simulink model "Rotating"  (R2023a)
settings: Solver=VariableStepAuto  StartTime=0.0  StopTime=40  RelTol=1e-3
values from neighbouring files (symbols this model uses):
  Kd = 0.5    [FFFB_PosForce_ME.m]    (also in FFFB_PosForce_ME1.m = 2.8284; FFFB_PosForce_ME2.m = 2.8284; FFFB_Posarbitary_actual_Mass.m = 2.8284; FFFB_arbitary_actual_Mass.m = 2.8284)
  Ki = 0.1    [FFFB_PosForce_ME.m]
  Kp = 16    [FFFB_PosForce_ME.m]    (also in FFFB_PosForce_ME1.m = 2; FFFB_PosForce_ME2.m = 2; FFFB_Posarbitary_actual_Mass.m = 2; FFFB_arbitary_actual_Mass.m = 2)
  N = [-y1+y3;-x3+x1]    [Contact.m]
  X = 0.65    [Contact.m]    (also in FFFB_PosForce_ME.m = [X0',X1',X2']; FFFB_PosForce_ME1.m = [X2']; FFFB_PosForce_ME2.m = [X110,X2']; FFFB_Posarbitary_actual_Mass.m = [X110])
  Y = [Y0',Y1',Y2']    [FFFB_PosForce_ME.m]    (also in FFFB_PosForce_ME1.m = [Y2']; FFFB_PosForce_ME2.m = [Y110,Y2']; FFFB_Posarbitary_actual_Mass.m = [Y110]; FFFB_arbitary_actual_Mass.m = [Y2'])
undefined symbols (not defined in the file or in its folder): Z
libraries: sm_lib x24, nesl_utility x8, robotcorelib x1
settings Model: Creator=91996  LastModifiedBy=91996

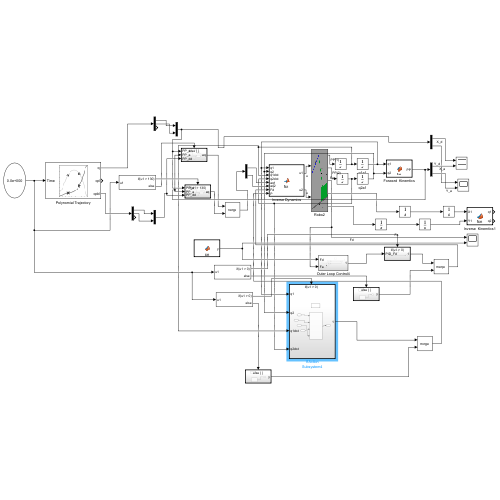
[thumbnail: Simulink's stored preview of the top-level diagram]
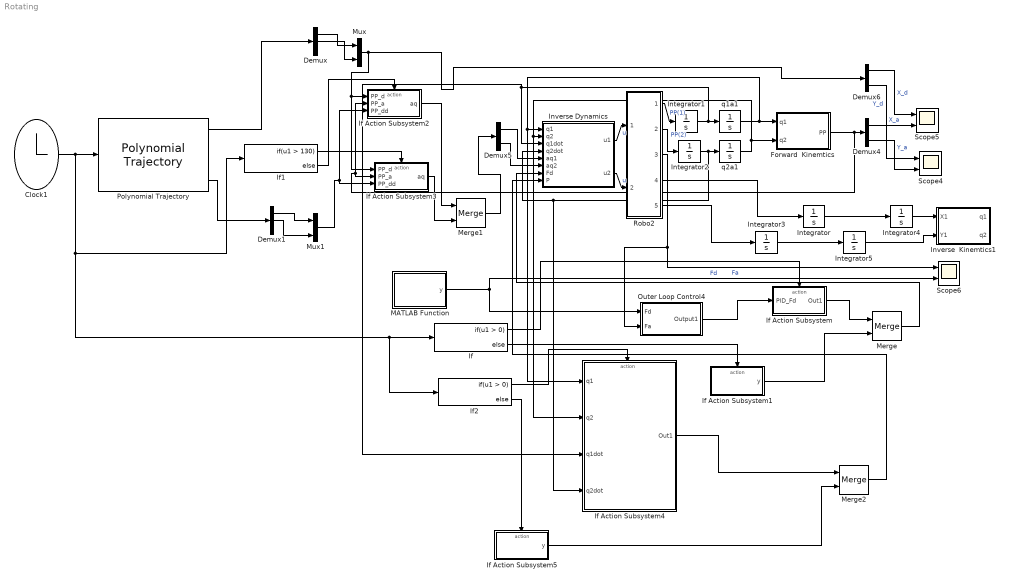
== system Rotating ==
  Clock1 : Clock
  Demux : Demux  Outputs=3
  Demux1 : Demux  Outputs=3
  Demux4 : Demux  Outputs=2
  Demux5 : Demux  Outputs=2
  Demux6 : Demux  Outputs=2
  Forward  Kinemtics : MATLAB Function  TreatAsAtomicUnit=on
  If : If
  If Action Subsystem : Subsystem  TreatAsAtomicUnit=on
  If Action Subsystem1 : Subsystem  TreatAsAtomicUnit=on
  If Action Subsystem2 : Subsystem  TreatAsAtomicUnit=on
  If Action Subsystem3 : Subsystem  TreatAsAtomicUnit=on
  If Action Subsystem4 : Subsystem  TreatAsAtomicUnit=on
  If Action Subsystem5 : Subsystem  TreatAsAtomicUnit=on
  If1 : If  IfExpression=u1 > 130
  If2 : If
  Integrator{,1..5} (6 alike) : Integrator
  Inverse  Kinemtics1 : MATLAB Function  TreatAsAtomicUnit=on
  Inverse Dynamics : MATLAB Function  TreatAsAtomicUnit=on
  MATLAB Function : MATLAB Function  TreatAsAtomicUnit=on
  Merge : Merge
  Merge1 : Merge
  Merge2 : Merge
  Mux : Mux  Inputs=2
  Mux1 : Mux  Inputs=2
  Outer Loop Control4 : Subsystem
  Polynomial Trajectory : robotcorelib/Polynomial Trajectory  WaypointSource=Internal  Waypoints=P  TimePoints=T  TimeInterval=[ 1, 4 ]  Method=Quintic Polynomial  ParameterSource=Internal  VelocityBoundaryCondition=Pd  AccelerationBoundaryCondition=Pdd  SimulateUsing=Interpreted execution
  Robo2 : Subsystem
      mask Display: image('C:\Users\91996\Desktop\2R-Robot Manipultor.png'); % Use "Edit Image" on toolstrip to change.
  Scope4 : Scope  NumInputPorts=2
  Scope5 : Scope  NumInputPorts=2
  Scope6 : Scope  NumInputPorts=2
  q1a1 : Integrator  InitialCondition=0.3330
  q2a1 : Integrator  InitialCondition=-1.5195
  wires:
  Inverse Dynamics/1(u1) -> Robo2/1(Input)  "u"
  Polynomial Trajectory/1 -> Demux/1
  Demux5/2 -> Inverse Dynamics/6(aq2)
  Demux6/2 -> Scope4/1  "Y_d"
  Mux/1 -> If Action Subsystem3/1(PP_d), If Action Subsystem2/1(PP_d), Demux6/1
  Demux1/2 -> Mux1/2
  Integrator4/1 -> Inverse  Kinemtics1/1(X1)
  Robo2/5(Y_dd) -> Integrator3/1
  Demux/1 -> Mux/1
  Integrator/1 -> Integrator4/1
  If2/1 -> If Action Subsystem4/Action
  Integrator3/1 -> Integrator5/1
  Demux1/1 -> Mux1/1
  Integrator5/1 -> Inverse  Kinemtics1/2(Y1)
  Demux5/1 -> Inverse Dynamics/5(aq1)
  Mux1/1 -> If Action Subsystem2/3(PP_dd), If Action Subsystem3/3(PP_dd)
  Polynomial Trajectory/3 -> Demux1/1
  If1/2 -> If Action Subsystem2/Action
  Demux4/1 -> Scope5/2  "X_a"
  Robo2/3(Output2) -> Scope6/1, Outer Loop Control4/2(Fa)  "Fa"
  If/1 -> If Action Subsystem/Action
  If Action Subsystem2/1(aq) -> Merge1/1
  If1/1 -> If Action Subsystem3/Action
  If Action Subsystem/1(Out1) -> Merge/1
  Merge1/1 -> Demux5/1
  Clock1/1 -> Polynomial Trajectory/1, If1/1, If2/1, If/1
  q2a1/1 -> If Action Subsystem4/2(q2), Inverse Dynamics/2(q2), Forward  Kinemtics/2(q2)
  Outer Loop Control4/1(Output1) -> If Action Subsystem/1(PID_Fd)
  If Action Subsystem3/1(aq) -> Merge1/2
  Forward  Kinemtics/1(PP) -> If Action Subsystem3/2(PP_a), If Action Subsystem2/2(PP_a), Demux4/1
  If Action Subsystem5/1(y) -> Merge2/2
  Merge2/1 -> Inverse Dynamics/8(P)
  MATLAB Function/1(y) -> Scope6/2, Outer Loop Control4/1(Fd)  "Fd"
  Robo2/4(X_dd) -> Integrator/1
  Merge/1 -> Inverse Dynamics/7(Fd)
  Integrator2/1 -> Inverse Dynamics/4(q2dot), If Action Subsystem4/4(q2dot), q2a1/1
  If Action Subsystem4/1(Out1) -> Merge2/1
  If2/2 -> If Action Subsystem5/Action
  Demux6/1 -> Scope5/1  "X_d"
  Inverse Dynamics/2(u2) -> Robo2/2(Input1)  "u"
  Integrator1/1 -> If Action Subsystem4/3(q1dot), Inverse Dynamics/3(q1dot), q1a1/1
  Robo2/2(q2_dd) -> Integrator2/1  "PP(2)"
  q1a1/1 -> Forward  Kinemtics/1(q1), If Action Subsystem4/1(q1), Inverse Dynamics/1(q1)
  Robo2/1(q1_dd) -> Integrator1/1  "PP(1)"
  If/2 -> If Action Subsystem1/Action
  Demux/2 -> Mux/2
  Demux4/2 -> Scope4/2  "Y_a"
  If Action Subsystem1/1(y) -> Merge/2

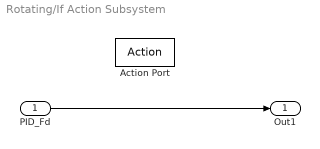
== system Rotating/If Action Subsystem ==
  PID_Fd : Inport
  Action Port : ActionPort  ActionPortLabel=if(u1 > 0)
  Out1 : Outport
  wires:
  PID_Fd/1 -> Out1/1

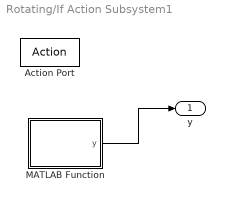
== system Rotating/If Action Subsystem1 ==
  Action Port : ActionPort  ActionPortLabel=else
  MATLAB Function : MATLAB Function  TreatAsAtomicUnit=on
  y : Outport
  wires:
  MATLAB Function/1(y) -> y/1

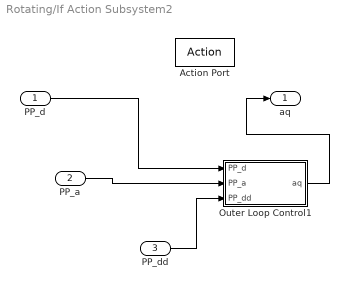
== system Rotating/If Action Subsystem2 ==
  PP_d : Inport
  PP_a : Inport  Port=2
  PP_dd : Inport  Port=3
  Action Port : ActionPort  ActionPortLabel=else
  Outer Loop Control1 : Subsystem
  aq : Outport
  wires:
  PP_d/1 -> Outer Loop Control1/1(PP_d)
  PP_dd/1 -> Outer Loop Control1/3(PP_dd)
  Outer Loop Control1/1(aq) -> aq/1
  PP_a/1 -> Outer Loop Control1/2(PP_a)

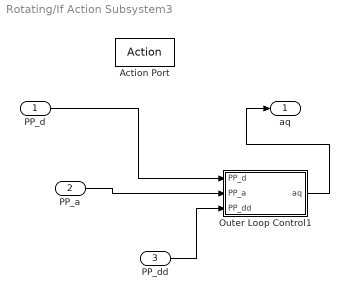
== system Rotating/If Action Subsystem3 ==
  PP_d : Inport
  PP_a : Inport  Port=2
  PP_dd : Inport  Port=3
  Action Port : ActionPort  ActionPortLabel=if(u1 > 130)
  Outer Loop Control1 : Subsystem
  aq : Outport
  wires:
  Outer Loop Control1/1(aq) -> aq/1
  PP_dd/1 -> Outer Loop Control1/3(PP_dd)
  PP_a/1 -> Outer Loop Control1/2(PP_a)
  PP_d/1 -> Outer Loop Control1/1(PP_d)

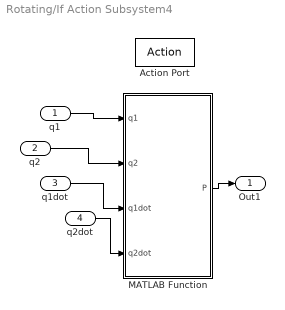
== system Rotating/If Action Subsystem4 ==
  q1 : Inport
  q2 : Inport  Port=2
  q1dot : Inport  Port=3
  q2dot : Inport  Port=4
  Action Port : ActionPort  ActionPortLabel=if(u1 > 0)
  MATLAB Function : MATLAB Function  TreatAsAtomicUnit=on
  Out1 : Outport
  wires:
  MATLAB Function/1(P) -> Out1/1
  q1/1 -> MATLAB Function/1(q1)
  q2/1 -> MATLAB Function/2(q2)
  q1dot/1 -> MATLAB Function/3(q1dot)
  q2dot/1 -> MATLAB Function/4(q2dot)

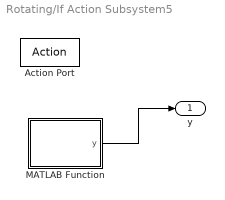
== system Rotating/If Action Subsystem5 ==
  Action Port : ActionPort  ActionPortLabel=else
  MATLAB Function : MATLAB Function  TreatAsAtomicUnit=on
  y : Outport
  wires:
  MATLAB Function/1(y) -> y/1

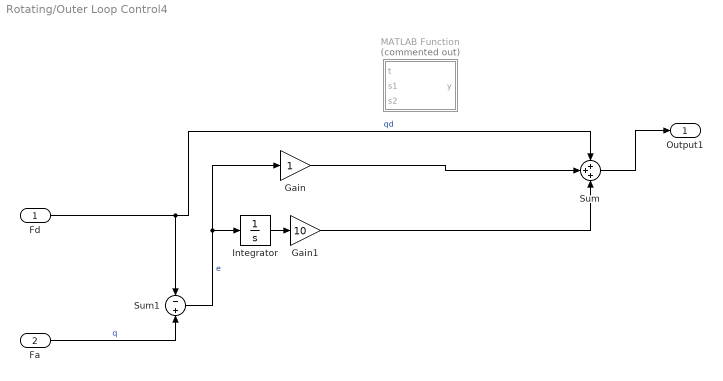
== system Rotating/Outer Loop Control4 ==
  Fd : Inport
  Fa : Inport  Port=2
  Gain : Gain
  Gain1 : Gain  Gain=10
  Integrator : Integrator
  MATLAB Function : MATLAB Function  Commented=on  TreatAsAtomicUnit=on
  Sum : Sum  Inputs=+++
  Sum1 : Sum  Inputs=-+
  Output1 : Outport
  wires:
  Sum1/1 -> Gain/1, Integrator/1  "e"
  Fd/1 -> Sum/1, Sum1/1  "qd"
  Fa/1 -> Sum1/2  "q"
  Integrator/1 -> Gain1/1
  Gain/1 -> Sum/2
  Gain1/1 -> Sum/3
  Sum/1 -> Output1/1

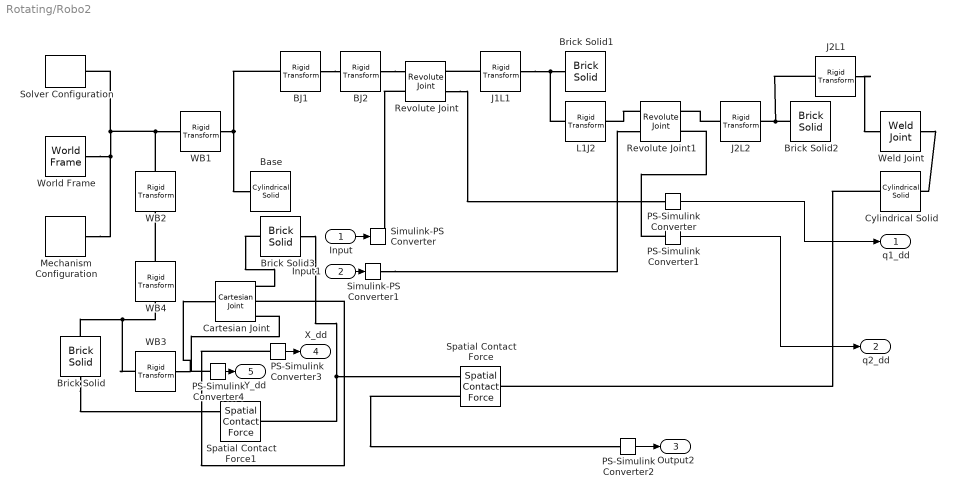
== system Rotating/Robo2 ==
  Input : Inport
  Input1 : Inport  Port=2
  BJ1 : sm_lib/Frames and Transforms/Rigid Transform  TranslationMethod=StandardAxis  TranslationStandardOffset=0.25  TranslationStandardOffsetUnits=m  TranslationStandardAxis=+Z  TranslationCartesianOffset=[0 0 0]  TranslationCartesianOffsetUnits=m  TranslationROffset=0  TranslationROffsetUnits=m  TranslationZOffset=0  TranslationZOffsetUnits=m  TranslationThetaOffset=0  TranslationThetaOffsetUnits=deg  RotationMethod=StandardAxis  RotationAngleUnits=deg  RotationStandardAxis=+X  RotationAngle=90  RotationArbitraryAxis=[0 0 1]  FollAlignAxisA=+X  BaseAlignAxisA=+Y  FollAlignAxisB=+Y  BaseAlignAxisB=+Z  RotationSequenceAxes=FollowerAxes  RotationSequence=XYX  RotationSequenceAngles=[0 0 0]  RotationSequenceAnglesUnits=deg  RotationMatrix=[1 0 0; 0 1 0; 0 0 1]  Quaternion=[1 0 0 0]
  BJ2 : sm_lib/Frames and Transforms/Rigid Transform  TranslationMethod=None  TranslationStandardOffset=0  TranslationStandardOffsetUnits=m  TranslationStandardAxis=+Z  TranslationCartesianOffset=[0 0 0]  TranslationCartesianOffsetUnits=m  TranslationROffset=0  TranslationROffsetUnits=m  TranslationZOffset=0  TranslationZOffsetUnits=m  TranslationThetaOffset=0  TranslationThetaOffsetUnits=deg  RotationMethod=StandardAxis  RotationAngleUnits=rad  RotationStandardAxis=+Z  RotationAngle=0.3330  RotationArbitraryAxis=[0 0 1]  FollAlignAxisA=+X  BaseAlignAxisA=+Y  FollAlignAxisB=+Y  BaseAlignAxisB=+Z  RotationSequenceAxes=FollowerAxes  RotationSequence=XYX  RotationSequenceAngles=[0 0 0]  RotationSequenceAnglesUnits=deg  RotationMatrix=[1 0 0; 0 1 0; 0 0 1]  Quaternion=[1 0 0 0]
  Base : sm_lib/Body Elements/Cylindrical Solid  GraphicAmbientColor=[0.15 0.15 0.15 1.0]  BasedOnType=Density  CenterOfMass=[0 0 0]  CenterOfMassUnits=m  GraphicDiffuseColor=[0.5 0.5 0.5]  CylinderLength=0.5  CylinderLengthUnits=m  CylinderRadius=0.02  CylinderRadiusUnits=m  Density=10000  DensityUnits=kg/m^3  DoExposeReferenceFrame=on  GraphicEmissiveColor=[0.0 0.0 0.0 1.0]  ExportEntireGeometry=off  SerializedFrames=<Frames/>  MarkerShape=Sphere  MarkerSize=10  GraphicType=FromGeometry  InertiaType=CalculateFromGeometry  Mass=1  MassUnits=kg  MomentsOfInertia=[1 1 1]  MomentsOfInertiaUnits=kg*m^2  GraphicOpacity=1.0  ProductsOfInertia=[0 0 0]  ProductsOfInertiaUnits=kg*m^2  GraphicShininess=75  GraphicSpecularColor=[0.5 0.5 0.5 1.0]  GraphicVisPropType=SimpleVisualProperties
  Brick Solid : sm_lib/Body Elements/Brick Solid  GraphicAmbientColor=[0.15 0.15 0.15 1.0]  BasedOnType=Density  BrickDimensions=[1 0.02 0.02]  BrickDimensionsUnits=m  CenterOfMass=[0 0 0]  CenterOfMassUnits=m  GraphicDiffuseColor=[0.5 0.5 0.5]  Density=10000  DensityUnits=kg/m^3  DoExposeReferenceFrame=on  GraphicEmissiveColor=[0.0 0.0 0.0 1.0]  ExportEntireGeometry=on  SerializedFrames=<Frames/>  MarkerShape=Sphere  MarkerSize=10  GraphicType=FromGeometry  InertiaType=CalculateFromGeometry  Mass=1  MassUnits=kg  MomentsOfInertia=[1 1 1]  MomentsOfInertiaUnits=kg*m^2  GraphicOpacity=1.0  ProductsOfInertia=[0 0 0]  ProductsOfInertiaUnits=kg*m^2  GraphicShininess=75  GraphicSpecularColor=[0.5 0.5 0.5 1.0]  GraphicVisPropType=SimpleVisualProperties
  Brick Solid1 : sm_lib/Body Elements/Brick Solid  GraphicAmbientColor=[0.15 0.15 0.15 1.0]  BasedOnType=Density  BrickDimensions=[0.5 0.02 0.02]  BrickDimensionsUnits=m  CenterOfMass=[0 0 0]  CenterOfMassUnits=m  GraphicDiffuseColor=[0.2 0.2 1.0]  Density=7800  DensityUnits=kg/m^3  DoExposeReferenceFrame=on  GraphicEmissiveColor=[0.0 0.0 0.0 1.0]  ExportEntireGeometry=off  SerializedFrames=<Frames/>  MarkerShape=Sphere  MarkerSize=10  GraphicType=FromGeometry  InertiaType=CalculateFromGeometry  Mass=1  MassUnits=kg  MomentsOfInertia=[1 1 1]  MomentsOfInertiaUnits=kg*m^2  GraphicOpacity=1.0  ProductsOfInertia=[0 0 0]  ProductsOfInertiaUnits=kg*m^2  GraphicShininess=75  GraphicSpecularColor=[0.5 0.5 0.5 1.0]  GraphicVisPropType=SimpleVisualProperties
  Brick Solid2 : sm_lib/Body Elements/Brick Solid  GraphicAmbientColor=[0.15 0.15 0.15 1.0]  BasedOnType=Density  BrickDimensions=[0.5-0.01 0.02 0.02]  BrickDimensionsUnits=m  CenterOfMass=[0 0 0]  CenterOfMassUnits=m  GraphicDiffuseColor=[0.0 0.8 0.2]  Density=7800  DensityUnits=kg/m^3  DoExposeReferenceFrame=on  GraphicEmissiveColor=[0.0 0.0 0.0 1.0]  ExportEntireGeometry=off  SerializedFrames=<Frames/>  MarkerShape=Sphere  MarkerSize=10  GraphicType=FromGeometry  InertiaType=CalculateFromGeometry  Mass=1  MassUnits=kg  MomentsOfInertia=[1 1 1]  MomentsOfInertiaUnits=kg*m^2  GraphicOpacity=1.0  ProductsOfInertia=[0 0 0]  ProductsOfInertiaUnits=kg*m^2  GraphicShininess=75  GraphicSpecularColor=[0.5 0.5 0.5 1.0]  GraphicVisPropType=SimpleVisualProperties
  Brick Solid3 : sm_lib/Body Elements/Brick Solid  GraphicAmbientColor=[0.15 0.15 0.15 1.0]  BasedOnType=Density  BrickDimensions=[0.2 0.02 0.2]  BrickDimensionsUnits=m  CenterOfMass=[0 0 0]  CenterOfMassUnits=m  GraphicDiffuseColor=[0.5 0.5 0.5]  Density=2000  DensityUnits=kg/m^3  DoExposeReferenceFrame=on  GraphicEmissiveColor=[0.0 0.0 0.0 1.0]  ExportEntireGeometry=on  SerializedFrames=<Frames/>  MarkerShape=Sphere  MarkerSize=10  GraphicType=FromGeometry  InertiaType=CalculateFromGeometry  Mass=1  MassUnits=kg  MomentsOfInertia=[1 1 1]  MomentsOfInertiaUnits=kg*m^2  GraphicOpacity=1.0  ProductsOfInertia=[0 0 0]  ProductsOfInertiaUnits=kg*m^2  GraphicShininess=75  GraphicSpecularColor=[0.5 0.5 0.5 1.0]  GraphicVisPropType=SimpleVisualProperties
  Cartesian Joint : sm_lib/Joints/Cartesian Joint  JointMode=Normal  SenseConstraintForce=off  SenseConstraintForceX=off  SenseConstraintForceY=off  SenseConstraintForceZ=off  SenseConstraintTorque=off  SenseConstraintTorqueX=off  SenseConstraintTorqueY=off  SenseConstraintTorqueZ=off  SenseTotalForce=off  SenseTotalForceX=off  SenseTotalForceY=off  SenseTotalForceZ=off  SenseTotalTorque=off  SenseTotalTorqueX=off  SenseTotalTorqueY=off  SenseTotalTorqueZ=off  CompositeWrenchDir=FollowerOnBase  CompositeWrenchFrame=BaseFrame  PxEquilibriumPosition=0  PxEquilibriumPositionUnits=m  PxSpringStiffness=0  PxSpringStiffnessUnits=N/m  PxDampingCoefficient=0  PxDampingCoefficientUnits=N/(m/s)  PxTorqueActuationMode=NoTorque  PxMotionActuationMode=ComputedMotion  PxSensePosition=off  PxSenseVelocity=off  PxSenseAcceleration=on  PxSenseTorqueForce=off  PxSenseLowerLimitTorqueForce=off  PxSenseUpperLimitTorqueForce=off  PxLowerLimitSpecify=off  PxLowerLimitBound=-1  PxLowerLimitBoundUnits=m  PxLowerLimitStiffness=1e6  PxLowerLimitStiffnessUnits=N/m  PxLowerLimitDamping=1e3  PxLowerLimitDampingUnits=N/(m/s)  PxLowerLimitTransitionRegionWidth=1e-4  PxLowerLimitTransitionRegionWidthUnits=m  PxUpperLimitSpecify=off  PxUpperLimitBound=1  PxUpperLimitBoundUnits=m  PxUpperLimitStiffness=1e6  PxUpperLimitStiffnessUnits=N/m  PxUpperLimitDamping=1e3  PxUpperLimitDampingUnits=N/(m/s)  PxUpperLimitTransitionRegionWidth=1e-4  PxUpperLimitTransitionRegionWidthUnits=m  PxPositionTargetSpecify=off  PxPositionTargetPriority=High  PxPositionTargetValue=0  PxPositionTargetValueUnits=m  PxVelocityTargetSpecify=off  PxVelocityTargetPriority=High  PxVelocityTargetValue=0  PxVelocityTargetValueUnits=m/s  PyEquilibriumPosition=0  PyEquilibriumPositionUnits=m  PySpringStiffness=0  PySpringStiffnessUnits=N/m  PyDampingCoefficient=0  PyDampingCoefficientUnits=N/(m/s)  PyTorqueActuationMode=NoTorque  PyMotionActuationMode=ComputedMotion  PySensePosition=off  PySenseVelocity=off  PySenseAcceleration=off  PySenseTorqueForce=off  PySenseLowerLimitTorqueForce=off  PySenseUpperLimitTorqueForce=off  PyLowerLimitSpecify=off  PyLowerLimitBound=-1  PyLowerLimitBoundUnits=m  PyLowerLimitStiffness=1e6  PyLowerLimitStiffnessUnits=N/m  PyLowerLimitDamping=1e3  PyLowerLimitDampingUnits=N/(m/s)  PyLowerLimitTransitionRegionWidth=1e-4  PyLowerLimitTransitionRegionWidthUnits=m  PyUpperLimitSpecify=off  PyUpperLimitBound=1  PyUpperLimitBoundUnits=m  PyUpperLimitStiffness=1e6  PyUpperLimitStiffnessUnits=N/m  PyUpperLimitDamping=1e3  PyUpperLimitDampingUnits=N/(m/s)  PyUpperLimitTransitionRegionWidth=1e-4  PyUpperLimitTransitionRegionWidthUnits=m  PyPositionTargetSpecify=off  PyPositionTargetPriority=High  PyPositionTargetValue=0  PyPositionTargetValueUnits=m  PyVelocityTargetSpecify=off  PyVelocityTargetPriority=High  PyVelocityTargetValue=0  PyVelocityTargetValueUnits=m/s  PzEquilibriumPosition=0  PzEquilibriumPositionUnits=m  PzSpringStiffness=0  PzSpringStiffnessUnits=N/m  PzDampingCoefficient=0  PzDampingCoefficientUnits=N/(m/s)  PzTorqueActuationMode=NoTorque  PzMotionActuationMode=ComputedMotion  PzSensePosition=off  PzSenseVelocity=off  PzSenseAcceleration=on  PzSenseTorqueForce=off  PzSenseLowerLimitTorqueForce=off  PzSenseUpperLimitTorqueForce=off  PzLowerLimitSpecify=off  PzLowerLimitBound=-1  PzLowerLimitBoundUnits=m  PzLowerLimitStiffness=1e6  PzLowerLimitStiffnessUnits=N/m  PzLowerLimitDamping=1e3  PzLowerLimitDampingUnits=N/(m/s)  PzLowerLimitTransitionRegionWidth=1e-4  PzLowerLimitTransitionRegionWidthUnits=m  PzUpperLimitSpecify=off  PzUpperLimitBound=1  PzUpperLimitBoundUnits=m  PzUpperLimitStiffness=1e6  PzUpperLimitStiffnessUnits=N/m  PzUpperLimitDamping=1e3  PzUpperLimitDampingUnits=N/(m/s)  PzUpperLimitTransitionRegionWidth=1e-4  PzUpperLimitTransitionRegionWidthUnits=m  PzPositionTargetSpecify=off  PzPositionTargetPriority=High  PzPositionTargetValue=0  PzPositionTargetValueUnits=m  PzVelocityTargetSpecify=off  PzVelocityTargetPriority=High  PzVelocityTargetValue=0  PzVelocityTargetValueUnits=m/s
  Cylindrical Solid : sm_lib/Body Elements/Cylindrical Solid  GraphicAmbientColor=[0.15 0.15 0.15 1.0]  BasedOnType=Density  CenterOfMass=[0 0 0]  CenterOfMassUnits=m  GraphicDiffuseColor=[0.5 0.5 0.5]  CylinderLength=0.02  CylinderLengthUnits=m  CylinderRadius=0.01  CylinderRadiusUnits=m  Density=7800  DensityUnits=kg/m^3  DoExposeReferenceFrame=on  GraphicEmissiveColor=[0.0 0.0 0.0 1.0]  ExportEntireGeometry=on  SerializedFrames=<Frames/>  MarkerShape=Sphere  MarkerSize=10  GraphicType=FromGeometry  InertiaType=CalculateFromGeometry  Mass=1  MassUnits=kg  MomentsOfInertia=[1 1 1]  MomentsOfInertiaUnits=kg*m^2  GraphicOpacity=1.0  ProductsOfInertia=[0 0 0]  ProductsOfInertiaUnits=kg*m^2  GraphicShininess=75  GraphicSpecularColor=[0.5 0.5 0.5 1.0]  GraphicVisPropType=SimpleVisualProperties
  J1L1 : sm_lib/Frames and Transforms/Rigid Transform  TranslationMethod=StandardAxis  TranslationStandardOffset=0.25  TranslationStandardOffsetUnits=m  TranslationStandardAxis=+X  TranslationCartesianOffset=[0 0 0]  TranslationCartesianOffsetUnits=m  TranslationROffset=0  TranslationROffsetUnits=m  TranslationZOffset=0  TranslationZOffsetUnits=m  TranslationThetaOffset=0  TranslationThetaOffsetUnits=deg  RotationMethod=None  RotationAngleUnits=deg  RotationStandardAxis=+Z  RotationAngle=0.0  RotationArbitraryAxis=[0 0 1]  FollAlignAxisA=+X  BaseAlignAxisA=+Y  FollAlignAxisB=+Y  BaseAlignAxisB=+Z  RotationSequenceAxes=FollowerAxes  RotationSequence=XYX  RotationSequenceAngles=[0 0 0]  RotationSequenceAnglesUnits=deg  RotationMatrix=[1 0 0; 0 1 0; 0 0 1]  Quaternion=[1 0 0 0]
  J2L1 : sm_lib/Frames and Transforms/Rigid Transform  TranslationMethod=StandardAxis  TranslationStandardOffset=(0.5-0.01)/2  TranslationStandardOffsetUnits=m  TranslationStandardAxis=+X  TranslationCartesianOffset=[0 0 0]  TranslationCartesianOffsetUnits=m  TranslationROffset=0  TranslationROffsetUnits=m  TranslationZOffset=0  TranslationZOffsetUnits=m  TranslationThetaOffset=0  TranslationThetaOffsetUnits=deg  RotationMethod=None  RotationAngleUnits=deg  RotationStandardAxis=+Z  RotationAngle=0.0  RotationArbitraryAxis=[0 0 1]  FollAlignAxisA=+X  BaseAlignAxisA=+Y  FollAlignAxisB=+Y  BaseAlignAxisB=+Z  RotationSequenceAxes=FollowerAxes  RotationSequence=XYX  RotationSequenceAngles=[0 0 0]  RotationSequenceAnglesUnits=deg  RotationMatrix=[1 0 0; 0 1 0; 0 0 1]  Quaternion=[1 0 0 0]
  J2L2 : sm_lib/Frames and Transforms/Rigid Transform  TranslationMethod=StandardAxis  TranslationStandardOffset=(0.5-0.01)/2  TranslationStandardOffsetUnits=m  TranslationStandardAxis=+X  TranslationCartesianOffset=[0 0 0]  TranslationCartesianOffsetUnits=m  TranslationROffset=0  TranslationROffsetUnits=m  TranslationZOffset=0  TranslationZOffsetUnits=m  TranslationThetaOffset=0  TranslationThetaOffsetUnits=deg  RotationMethod=None  RotationAngleUnits=deg  RotationStandardAxis=+Z  RotationAngle=0.0  RotationArbitraryAxis=[0 0 1]  FollAlignAxisA=+X  BaseAlignAxisA=+Y  FollAlignAxisB=+Y  BaseAlignAxisB=+Z  RotationSequenceAxes=FollowerAxes  RotationSequence=XYX  RotationSequenceAngles=[0 0 0]  RotationSequenceAnglesUnits=deg  RotationMatrix=[1 0 0; 0 1 0; 0 0 1]  Quaternion=[1 0 0 0]
  L1J2 : sm_lib/Frames and Transforms/Rigid Transform  TranslationMethod=StandardAxis  TranslationStandardOffset=0.25  TranslationStandardOffsetUnits=m  TranslationStandardAxis=+X  TranslationCartesianOffset=[0 0 0]  TranslationCartesianOffsetUnits=m  TranslationROffset=0  TranslationROffsetUnits=m  TranslationZOffset=0  TranslationZOffsetUnits=m  TranslationThetaOffset=0  TranslationThetaOffsetUnits=deg  RotationMethod=StandardAxis  RotationAngleUnits=rad  RotationStandardAxis=+Z  RotationAngle=-1.5195  RotationArbitraryAxis=[0 0 1]  FollAlignAxisA=+X  BaseAlignAxisA=+Y  FollAlignAxisB=+Y  BaseAlignAxisB=+Z  RotationSequenceAxes=FollowerAxes  RotationSequence=XYX  RotationSequenceAngles=[0 0 0]  RotationSequenceAnglesUnits=deg  RotationMatrix=[1 0 0; 0 1 0; 0 0 1]  Quaternion=[1 0 0 0]
  Mechanism Configuration : sm_lib/Utilities/Mechanism Configuration  UniformGravity=Constant  GravityVector=[0 0 -9.80665]  GravityVectorUnits=m/s^2  LinearizationDelta=0.001  JointModeTransitionNonlinearIterations=2
  PS-Simulink Converter{,1..4} (5 alike) : nesl_utility/PS-Simulink Converter  PhysicalDomain=network_engine_domain  SubClassName=ps_output  LeftPortType=input  RightPortType=output  PseudoPeriodic=off  Frequencies=[]  VectorFormat=inherit  Unit=inherit  AffineConversion=off
  Revolute Joint : sm_lib/Joints/Revolute Joint  JointMode=Normal  SenseConstraintForce=off  SenseConstraintForceX=off  SenseConstraintForceY=off  SenseConstraintForceZ=off  SenseConstraintTorque=off  SenseConstraintTorqueX=off  SenseConstraintTorqueY=off  SenseConstraintTorqueZ=off  SenseTotalForce=off  SenseTotalForceX=off  SenseTotalForceY=off  SenseTotalForceZ=off  SenseTotalTorque=off  SenseTotalTorqueX=off  SenseTotalTorqueY=off  SenseTotalTorqueZ=off  CompositeWrenchDir=FollowerOnBase  CompositeWrenchFrame=BaseFrame  EquilibriumPosition=0  EquilibriumPositionUnits=deg  SpringStiffness=0  SpringStiffnessUnits=N*m/deg  DampingCoefficient=0  DampingCoefficientUnits=N*m/(deg/s)  TorqueActuationMode=InputTorque  MotionActuationMode=ComputedMotion  SensePosition=off  SenseVelocity=off  SenseAcceleration=on  SenseTorqueForce=off  SenseLowerLimitTorqueForce=off  SenseUpperLimitTorqueForce=off  LowerLimitSpecify=off  LowerLimitBound=-90  LowerLimitBoundUnits=deg  LowerLimitStiffness=1e4  LowerLimitStiffnessUnits=N*m/deg  LowerLimitDamping=10  LowerLimitDampingUnits=N*m/(deg/s)  LowerLimitTransitionRegionWidth=0.1  LowerLimitTransitionRegionWidthUnits=deg  UpperLimitSpecify=off  UpperLimitBound=90  UpperLimitBoundUnits=deg  UpperLimitStiffness=1e4  UpperLimitStiffnessUnits=N*m/deg  UpperLimitDamping=10  UpperLimitDampingUnits=N*m/(deg/s)  UpperLimitTransitionRegionWidth=0.1  UpperLimitTransitionRegionWidthUnits=deg  PositionTargetSpecify=off  PositionTargetPriority=High  PositionTargetValue=0  PositionTargetValueUnits=deg  VelocityTargetSpecify=off  VelocityTargetPriority=High  VelocityTargetValue=0  VelocityTargetValueUnits=deg/s
  Revolute Joint1 : sm_lib/Joints/Revolute Joint  JointMode=Normal  SenseConstraintForce=off  SenseConstraintForceX=off  SenseConstraintForceY=off  SenseConstraintForceZ=off  SenseConstraintTorque=off  SenseConstraintTorqueX=off  SenseConstraintTorqueY=off  SenseConstraintTorqueZ=off  SenseTotalForce=off  SenseTotalForceX=off  SenseTotalForceY=off  SenseTotalForceZ=off  SenseTotalTorque=off  SenseTotalTorqueX=off  SenseTotalTorqueY=off  SenseTotalTorqueZ=off  CompositeWrenchDir=FollowerOnBase  CompositeWrenchFrame=BaseFrame  EquilibriumPosition=0  EquilibriumPositionUnits=deg  SpringStiffness=0  SpringStiffnessUnits=N*m/deg  DampingCoefficient=0  DampingCoefficientUnits=N*m/(deg/s)  TorqueActuationMode=InputTorque  MotionActuationMode=ComputedMotion  SensePosition=off  SenseVelocity=off  SenseAcceleration=on  SenseTorqueForce=off  SenseLowerLimitTorqueForce=off  SenseUpperLimitTorqueForce=off  LowerLimitSpecify=off  LowerLimitBound=-90  LowerLimitBoundUnits=deg  LowerLimitStiffness=1e4  LowerLimitStiffnessUnits=N*m/deg  LowerLimitDamping=10  LowerLimitDampingUnits=N*m/(deg/s)  LowerLimitTransitionRegionWidth=0.1  LowerLimitTransitionRegionWidthUnits=deg  UpperLimitSpecify=off  UpperLimitBound=90  UpperLimitBoundUnits=deg  UpperLimitStiffness=1e4  UpperLimitStiffnessUnits=N*m/deg  UpperLimitDamping=10  UpperLimitDampingUnits=N*m/(deg/s)  UpperLimitTransitionRegionWidth=0.1  UpperLimitTransitionRegionWidthUnits=deg  PositionTargetSpecify=off  PositionTargetPriority=High  PositionTargetValue=0  PositionTargetValueUnits=deg  VelocityTargetSpecify=off  VelocityTargetPriority=High  VelocityTargetValue=0  VelocityTargetValueUnits=deg/s
  Simulink-PS Converter : nesl_utility/Simulink-PS Converter  PhysicalDomain=network_engine_domain  SubClassName=ps_input  LeftPortType=input  RightPortType=output  PseudoPeriodic=off  Frequencies=[]  NoiseDistribution=none  NoiseParameters=[]  Unit=N*m  AffineConversion=off  FilteringAndDerivatives=provide  SimscapeFilterOrder=1  InputFilterTimeConstant=0.001  UdotUserProvided=0
  Simulink-PS Converter1 : nesl_utility/Simulink-PS Converter  PhysicalDomain=network_engine_domain  SubClassName=ps_input  LeftPortType=input  RightPortType=output  PseudoPeriodic=off  Frequencies=[]  NoiseDistribution=none  NoiseParameters=[]  Unit=N*m  AffineConversion=off  FilteringAndDerivatives=provide  SimscapeFilterOrder=1  InputFilterTimeConstant=0.001  UdotUserProvided=0
  Solver Configuration : nesl_utility/Solver Configuration  PhysicalDomain=network_engine_domain  SubClassName=solver  LeftPortType=input  RightPortType=generic  Tones=[]  Harmonics=[]  SimulateNoise=off  Profile=off  UseLocalSampling=off  EnableSwitchedLinearOptims=on  FrequencyDomain=off  UseCCode=off  RelTol=0.001  AbsTol=1e-06  MinStep=1e-09  ToWorkspace=off  RevertToSquareIcSolve=off  NumHomotopyIterations=100  PhasorMode=off  PhasorModeNumHarmonics=1  ConsistencySolver=NEWTON_XTOL_AFTER_FTOL  IndexReductionMethod=DerivativeReplacement  DoDC=off  ResidualTolerance=1e-09  ConsistencyTolSource=GLOBAL  ConsistencyAbsTol=0.001  ConsistencyRelTol=0.001  ConsistencyTolFactor=0.001  UseLocalSolver=off  LocalSolverChoice=NE_BACKWARD_EULER_ADVANCER  ResolveIndetEquations=on  FunctionEvalNumThread=1  LocalSolverSampleTime=0.001  DoFixedCost=off  MaxNonlinIter=3  MaxModeIter=2  ComputeImpulses=off  ImpulseIterations=2  LinearAlgebra=Sparse  LinearAlgebraNumThread=0  EquationFormulation=NE_TIME_EF  DelaysMemoryBudget=1024  AutomaticFiltering=on  FilteringTimeConstant=0.001  PartitionStorageMethod=AS_NEEDED  PartitionMemoryBudget=1024  PartitionMethod=FAST
  Spatial Contact Force : sm_lib/Forces and Torques/Spatial Contact Force  SenseContactBaseRotation=off  SenseContactBaseTranslation=off  CoefficientOfDynamicFriction=0.3  CoefficientOfStaticFriction=0.5  NormalDamping=1e6  NormalDampingUnits=N/(m/s)  SenseContactSignal=off  NormalStiffness=1e6  NormalStiffnessUnits=N/m  FrictionalCriticalVelocity=1e-3  FrictionalCriticalVelocityUnits=m/s  ZeroCrossDetectContactStartAndEnd=off  SenseContactFollowerRotation=off  SenseContactFollowerTranslation=off  FrictionType=SmoothStickSlip  SenseFrictionalForceMagnitude=off  SenseNormalForceMagnitude=on  NormalForceType=SmoothSpringDamper  SenseNormalVelocity=off  SenseSeparationDistance=off  SenseTangentialVelocity=off  NormalTransitionRegionWidth=1e-4  NormalTransitionRegionWidthUnits=m
  Spatial Contact Force1 : sm_lib/Forces and Torques/Spatial Contact Force  SenseContactBaseRotation=off  SenseContactBaseTranslation=off  CoefficientOfDynamicFriction=0.05  CoefficientOfStaticFriction=0.1  NormalDamping=1e6  NormalDampingUnits=N/(m/s)  SenseContactSignal=off  NormalStiffness=1e6  NormalStiffnessUnits=N/m  FrictionalCriticalVelocity=1e-3  FrictionalCriticalVelocityUnits=m/s  ZeroCrossDetectContactStartAndEnd=off  SenseContactFollowerRotation=off  SenseContactFollowerTranslation=off  FrictionType=SmoothStickSlip  SenseFrictionalForceMagnitude=off  SenseNormalForceMagnitude=on  NormalForceType=SmoothSpringDamper  SenseNormalVelocity=off  SenseSeparationDistance=off  SenseTangentialVelocity=off  NormalTransitionRegionWidth=1e-4  NormalTransitionRegionWidthUnits=m
  WB1 : sm_lib/Frames and Transforms/Rigid Transform  TranslationMethod=Cartesian  TranslationStandardOffset=0  TranslationStandardOffsetUnits=m  TranslationStandardAxis=+Z  TranslationCartesianOffset=[0 0.25 0]  TranslationCartesianOffsetUnits=m  TranslationROffset=0  TranslationROffsetUnits=m  TranslationZOffset=0  TranslationZOffsetUnits=m  TranslationThetaOffset=0  TranslationThetaOffsetUnits=deg  RotationMethod=None  RotationAngleUnits=deg  RotationStandardAxis=+X  RotationAngle=90  RotationArbitraryAxis=[0 0 1]  FollAlignAxisA=+X  BaseAlignAxisA=+Y  FollAlignAxisB=+Y  BaseAlignAxisB=+Z  RotationSequenceAxes=FollowerAxes  RotationSequence=XYX  RotationSequenceAngles=[0 0 0]  RotationSequenceAnglesUnits=deg  RotationMatrix=[1 0 0; 0 1 0; 0 0 1]  Quaternion=[1 0 0 0]
  WB2 : sm_lib/Frames and Transforms/Rigid Transform  TranslationMethod=Cartesian  TranslationStandardOffset=0  TranslationStandardOffsetUnits=m  TranslationStandardAxis=+Z  TranslationCartesianOffset="[-0.5   -0.25  0.25 ]"  TranslationCartesianOffsetUnits=m  TranslationROffset=0  TranslationROffsetUnits=m  TranslationZOffset=0  TranslationZOffsetUnits=m  TranslationThetaOffset=0  TranslationThetaOffsetUnits=deg  RotationMethod=None  RotationAngleUnits=deg  RotationStandardAxis=+X  RotationAngle=90  RotationArbitraryAxis=[0 0 1]  FollAlignAxisA=+X  BaseAlignAxisA=+Y  FollAlignAxisB=+Y  BaseAlignAxisB=+Z  RotationSequenceAxes=FollowerAxes  RotationSequence=XYX  RotationSequenceAngles=[0 0 0]  RotationSequenceAnglesUnits=deg  RotationMatrix=[1 0 0; 0 1 0; 0 0 1]  Quaternion=[1 0 0 0]
  WB3 : sm_lib/Frames and Transforms/Rigid Transform  TranslationMethod=Cartesian  TranslationStandardOffset=0  TranslationStandardOffsetUnits=m  TranslationStandardAxis=+Z  TranslationCartesianOffset="[-0.25  0  -0.1-0.01 ]"  TranslationCartesianOffsetUnits=m  TranslationROffset=0  TranslationROffsetUnits=m  TranslationZOffset=0  TranslationZOffsetUnits=m  TranslationThetaOffset=0  TranslationThetaOffsetUnits=deg  RotationMethod=None  RotationAngleUnits=deg  RotationStandardAxis=+X  RotationAngle=90  RotationArbitraryAxis=[0 0 1]  FollAlignAxisA=+X  BaseAlignAxisA=+Y  FollAlignAxisB=+Y  BaseAlignAxisB=+Z  RotationSequenceAxes=FollowerAxes  RotationSequence=XYX  RotationSequenceAngles=[0 0 0]  RotationSequenceAnglesUnits=deg  RotationMatrix=[1 0 0; 0 1 0; 0 0 1]  Quaternion=[1 0 0 0]
  WB4 : sm_lib/Frames and Transforms/Rigid Transform  TranslationMethod=Cartesian  TranslationStandardOffset=0  TranslationStandardOffsetUnits=m  TranslationStandardAxis=+Z  TranslationCartesianOffset=[0,0,0.01 ]  TranslationCartesianOffsetUnits=m  TranslationROffset=0  TranslationROffsetUnits=m  TranslationZOffset=0  TranslationZOffsetUnits=m  TranslationThetaOffset=0  TranslationThetaOffsetUnits=deg  RotationMethod=None  RotationAngleUnits=deg  RotationStandardAxis=+X  RotationAngle=90  RotationArbitraryAxis=[0 0 1]  FollAlignAxisA=+X  BaseAlignAxisA=+Y  FollAlignAxisB=+Y  BaseAlignAxisB=+Z  RotationSequenceAxes=FollowerAxes  RotationSequence=XYX  RotationSequenceAngles=[0 0 0]  RotationSequenceAnglesUnits=deg  RotationMatrix=[1 0 0; 0 1 0; 0 0 1]  Quaternion=[1 0 0 0]
  Weld Joint : sm_lib/Joints/Weld Joint  JointMode=Normal  SenseConstraintForce=off  SenseConstraintForceX=off  SenseConstraintForceY=off  SenseConstraintForceZ=off  SenseConstraintTorque=off  SenseConstraintTorqueX=off  SenseConstraintTorqueY=off  SenseConstraintTorqueZ=off  SenseTotalForce=off  SenseTotalForceX=off  SenseTotalForceY=off  SenseTotalForceZ=off  SenseTotalTorque=off  SenseTotalTorqueX=off  SenseTotalTorqueY=off  SenseTotalTorqueZ=off  CompositeWrenchDir=FollowerOnBase  CompositeWrenchFrame=BaseFrame
  World Frame : sm_lib/Frames and Transforms/World Frame
  q1_dd : Outport
  q2_dd : Outport  Port=2
  Output2 : Outport  Port=3
  X_dd : Outport  Port=4
  Y_dd : Outport  Port=5
  wires:
  Input/1 -> Simulink-PS Converter/1
  Input1/1 -> Simulink-PS Converter1/1
  PS-Simulink Converter/1 -> q1_dd/1
  PS-Simulink Converter1/1 -> q2_dd/1
  PS-Simulink Converter2/1 -> Output2/1
  PS-Simulink Converter3/1 -> X_dd/1
  PS-Simulink Converter4/1 -> Y_dd/1
  connections:
  BJ1/LConn1 -- Base/RConn1 -- WB1/RConn1
  J1L1/RConn1 -- L1J2/LConn1 -- Brick Solid1/RConn1
  Revolute Joint1/LConn1 -- L1J2/RConn1
  Brick Solid2/RConn1 -- J2L1/LConn1 -- J2L2/RConn1
  J1L1/LConn1 -- Revolute Joint/RConn1
  J2L2/LConn1 -- Revolute Joint1/RConn1
  Revolute Joint/LConn2 -- Simulink-PS Converter/RConn1
  Simulink-PS Converter1/RConn1 -- Revolute Joint1/LConn2
  Revolute Joint/RConn2 -- PS-Simulink Converter/LConn1
  PS-Simulink Converter1/LConn1 -- Revolute Joint1/RConn2
  Solver Configuration/RConn1 -- WB2/RConn1 -- WB1/LConn1 -- Mechanism Configuration/RConn1 -- World Frame/RConn1
  WB4/RConn1 -- WB2/LConn1
  J2L1/RConn1 -- Weld Joint/LConn1
  Weld Joint/RConn1 -- Cylindrical Solid/RConn1
  BJ2/RConn1 -- Revolute Joint/LConn1
  WB4/LConn1 -- Brick Solid/RConn1 -- WB3/RConn1
  Spatial Contact Force/RConn2 -- PS-Simulink Converter2/LConn1
  BJ1/RConn1 -- BJ2/LConn1
  Brick Solid3/LConn1 -- Spatial Contact Force1/LConn1 -- Spatial Contact Force/RConn1
  Cylindrical Solid/LConn1 -- Spatial Contact Force/LConn1
  Brick Solid/LConn1 -- Spatial Contact Force1/RConn1
  WB3/LConn1 -- Cartesian Joint/LConn1
  Brick Solid3/RConn1 -- Cartesian Joint/RConn1
  PS-Simulink Converter3/LConn1 -- Cartesian Joint/RConn2
  PS-Simulink Converter4/LConn1 -- Cartesian Joint/RConn3

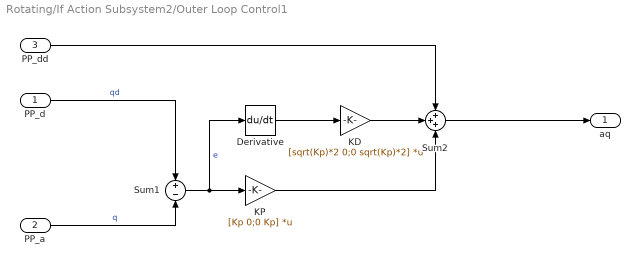
== system Rotating/If Action Subsystem2/Outer Loop Control1 ==
  PP_d : Inport
  PP_a : Inport  Port=2
  PP_dd : Inport  Port=3
  Derivative : Derivative
  KD : Gain  Gain=[sqrt(Kp)*2 0;0 sqrt(Kp)*2]  Multiplication=Matrix(K*u)
  KP : Gain  Gain=[Kp 0;0 Kp]  Multiplication=Matrix(K*u)
  Sum1 : Sum  Inputs=+-
  Sum2 : Sum  Inputs=+++
  aq : Outport
  wires:
  KD/1 -> Sum2/2
  KP/1 -> Sum2/3
  Sum1/1 -> Derivative/1, KP/1  "e"
  Derivative/1 -> KD/1
  PP_d/1 -> Sum1/1  "qd"
  PP_a/1 -> Sum1/2  "q"
  Sum2/1 -> aq/1
  PP_dd/1 -> Sum2/1

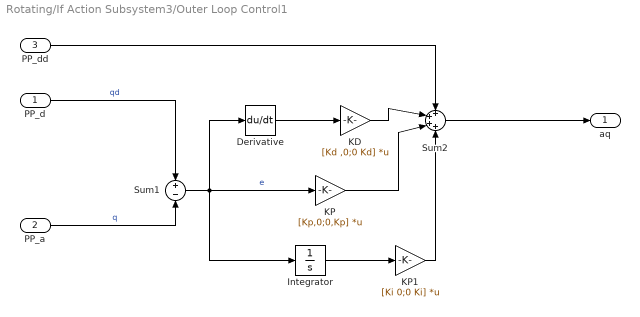
== system Rotating/If Action Subsystem3/Outer Loop Control1 ==
  PP_d : Inport
  PP_a : Inport  Port=2
  PP_dd : Inport  Port=3
  Derivative : Derivative
  Integrator : Integrator
  KD : Gain  Gain=[Kd ,0;0 Kd]  Multiplication=Matrix(K*u)
  KP : Gain  Gain=[Kp,0;0,Kp]  Multiplication=Matrix(K*u)
  KP1 : Gain  Gain=[Ki 0;0 Ki]  Multiplication=Matrix(K*u)
  Sum1 : Sum  Inputs=+-
  Sum2 : Sum  Inputs=++++
  aq : Outport
  wires:
  KD/1 -> Sum2/2
  KP/1 -> Sum2/3
  Sum1/1 -> Integrator/1, KP/1, Derivative/1  "e"
  Derivative/1 -> KD/1
  PP_d/1 -> Sum1/1  "qd"
  PP_a/1 -> Sum1/2  "q"
  Sum2/1 -> aq/1
  PP_dd/1 -> Sum2/1
  Integrator/1 -> KP1/1
  KP1/1 -> Sum2/4

== matlab function Rotating/Outer Loop Control4/MATLAB Function ==
  data: t input; y output; s1 input; s2 input
function y = fcn(t,s1,s2)
B=F0;

Kfp=0.01;
Kfi=-(Kfp)*log((s2/B))/(t+0.001);
y=real(s1*Kfi+s2*Kfi);

== matlab function Rotating/If Action Subsystem1/MATLAB Function ==
  data: y output
function y = fcn()

y = 0;

== matlab function Rotating/If Action Subsystem4/MATLAB Function ==
  data: q1 input; P output; q2 input; q1dot input; q2dot input
function P=  fcn(q1,q2,q1dot,q2dot)

g=9.81;
a1=0.5;  
a2=0.5; 
L01=0.5;
m1=1.56;
m2=1.5288;
m3=0.0490088;
C1=a1/2;
C2=(m2*0.5*a2+m3*a2)/(m2+m3);
Itot1=0.032552;
Itot2=0.0306397+2.45044e-06;
Jac = R_Jac1(a1,a2,q1,q2);
Jd=R_Jd1(a1,a2,q1,q2,q1dot,q2dot);
M=R_M(C1,C2,Itot1,Itot2,a1,m1,m2+m3,q2);
C =  R_damp(C2,a1,m2+m3,q2,q1dot,q2dot);
G= R_Gra(C1,C2,a1,m1,m2+m3,g,q1,q2);
Jac = R_Jac1(a1,a2,q1,q2);
Jd=R_Jd1(a1,a2,q1,q2,q1dot,q2dot);
mo=1.6;
Mo=[mo 0; 0 mo];
M_=inv(Jac')*M*inv(Jac)+Mo;
A =  [0, 1];
P=eye(2)-(A'*inv(A*inv(M_)*A')*A*inv(M_));

== matlab function Rotating/If Action Subsystem5/MATLAB Function ==
  data: y output
function y = fcn()

y = eye(2);

== matlab function Rotating/MATLAB Function ==
  data: y output
function y = fcn()

y =10;

== matlab function Rotating/Inverse  Kinemtics1 ==
  data: X1 input; q1 output; Y1 input; q2 output
function [q1,q2]= fcn(X1,Y1)
a1=0.5;
a2=0.5;
L01=0.5;
Z0=[1,2]';
for n=1:100
    q1=Z0(1);
    q2=Z0(2);
PP=R_EQ(L01,a1,a2,q1,q2)-[X1;Y1];
Jac = R_Jac1(a1,a2,q1,q2);

Z1=inv(Jac)*PP;
err=abs(Z1-Z0);
if err<=0.0001
    break
else Z0=Z1;
end
end

== matlab function Rotating/Inverse Dynamics ==
  data: q1 input; u1 output; q2 input; q1dot input; q2dot input; aq1 input; aq2 input; u2 output; Fd input; P input
function [u1,u2] = fcn(q1,q2,q1dot,q2dot,aq1,aq2,Fd,P)
% q2=q2-0.1;
g=9.81;
a1=0.5;  
a2=0.5; 
L01=0.5;
m1=1.56;
m2=1.5288;
m3=0.0490088;
C1=a1/2;
C2=(m2*0.5*a2+m3*a2)/(m2+m3);
Itot1=0.032552;
Itot2=0.0306397+2.45044e-06;
Jac = R_Jac1(a1,a2,q1,q2);
Jd=R_Jd1(a1,a2,q1,q2,q1dot,q2dot);
M=R_M(C1,C2,Itot1,Itot2,a1,m1,m2+m3,q2);
C = R_damp(C2,a1,m2+m3,q2,q1dot,q2dot);
G= R_Gra(C1,C2,a1,m1,m2+m3,g,q1,q2);
mo=1.6;
Mo=[mo 0; 0 0];
M_=inv(Jac')*M*inv(Jac)+Mo;
Fo=[mo*g*0.1;-mo*g]
nt=inv(Jac')*(-M*inv(Jac)*Jd*[q1dot;q1dot]+(C+G))+[0;mo*g]+Fo;
A =[0, 1];
u =Jac'*(P*(M_*[aq1;aq2]+nt)+(eye(2)-P)*(nt+A'*Fd));
u1=u(1);
u2=u(2);

== matlab function Rotating/Forward  Kinemtics ==
  data: q1 input; PP output; q2 input
function PP = fcn(q1,q2)
a1=0.5;
a2=0.5;
L01=0.5;
PP=R_EQ(L01,a1,a2,q1,q2);
